simulink library "environment_cl"  (R2018a)
settings: Solver=VariableStepAuto  StartTime=0.0  StopTime=10.0  RelTol=1e-3
libraries: flowVariants x1
settings Model: Creator=mitch  LastModifiedBy=mitch

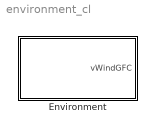
== system environment_cl ==
  Environment : Subsystem

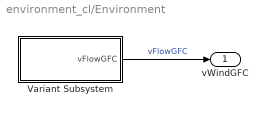
== system environment_cl/Environment ==
  Variant Subsystem : Subsystem  Variant=on
  vWindGFC : Outport
  wires:
  Variant Subsystem/1(vFlowGFC) -> vWindGFC/1  "vFlowGFC"

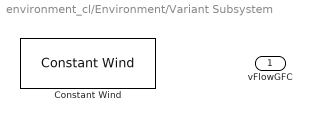
== system environment_cl/Environment/Variant Subsystem ==
  Constant Wind : flowVariants/Constant Wind  VariantControl=variantConstant
  vFlowGFC : Outport
